simulink model "untitled4"  (R2025a)
settings: Solver=VariableStepAuto  StartTime=0.0  StopTime=10.0  RelTol=1e-3
libraries: fuzblock x1
settings Model: Creator=Win 11  LastModifiedBy=Win 11

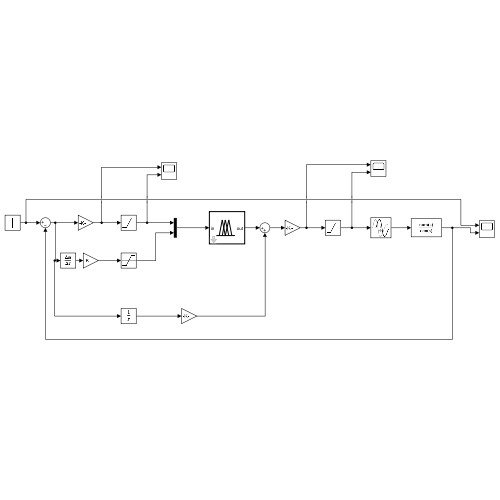
[thumbnail: Simulink's stored preview of the top-level diagram]
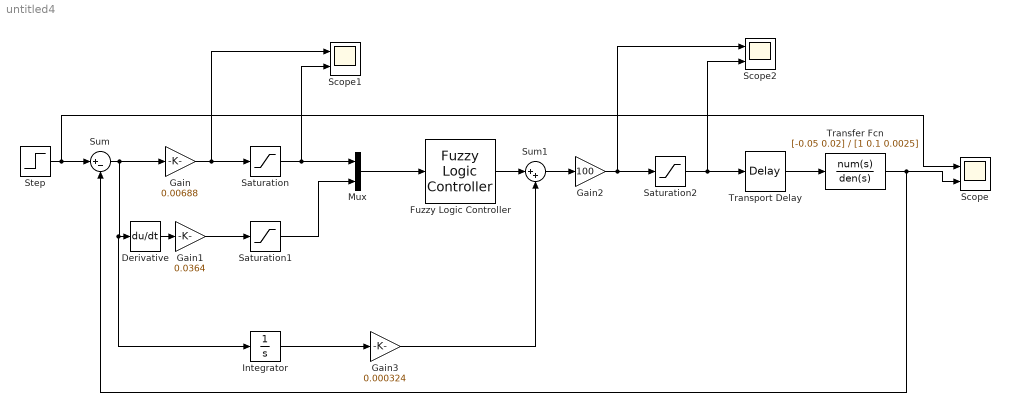
== system untitled4 ==
  Derivative : Derivative
  Fuzzy Logic Controller : fuzblock/Fuzzy Logic  Controller  FIS=fis  OutputSampleNumber=101  DataType=double  UseLookupTable=off  NumBreakpoints=10  FuzzifiedInputs=off  RuleFiringStrengths=off  RuleOutputs=off  AggregatedOutputs=off  SimulateUsing=Interpreted execution  OutOfRangeInputValueMessage=warning  NoRuleFiredMessage=warning  EmptyOutputFuzzySetMessage=warning
  Gain : Gain  Gain=0.00688
  Gain1 : Gain  Gain=0.0364
  Gain2 : Gain  Gain=100
  Gain3 : Gain  Gain=0.000324
  Integrator : Integrator
  Mux : Mux  Inputs=2
  Saturation : Saturate  UpperLimit=4  LowerLimit=-4
  Saturation1 : Saturate  UpperLimit=4  LowerLimit=-4
  Saturation2 : Saturate  UpperLimit=+2.2  LowerLimit=-2.2
  Scope : Scope  NumInputPorts=2
      settings: ActiveDisplayYMinimum=-0.140071912811771  ActiveDisplayYMaximum=1.1266746569790858
  Scope1 : Scope  NumInputPorts=2
      settings: ActiveDisplayYMinimum=-0.00087152164001610922  ActiveDisplayYMaximum=0.0078436947601449852
  Scope2 : Scope  NumInputPorts=2
      settings: ActiveDisplayYMinimum=-13.773649999999998  ActiveDisplayYMaximum=123.96285000000002  DataLoggingVariableName=ScopeData2
  Step : Step  SampleTime=0
  Sum : Sum  Inputs=|+-
  Sum1 : Sum  Inputs=|++
  Transfer Fcn : TransferFcn  Numerator=[-0.05 0.02]  Denominator=[1 0.1 0.0025]
  Transport Delay : TransportDelay  DelayTime=2
  wires:
  Step/1 -> Scope/1, Sum/1
  Gain/1 -> Scope1/1, Saturation/1
  Saturation/1 -> Scope1/2, Mux/1
  Saturation1/1 -> Mux/2
  Mux/1 -> Fuzzy Logic Controller/1
  Fuzzy Logic Controller/1 -> Sum1/1
  Sum1/1 -> Gain2/1
  Gain2/1 -> Scope2/1, Saturation2/1
  Saturation2/1 -> Scope2/2, Transport Delay/1
  Transport Delay/1 -> Transfer Fcn/1
  Transfer Fcn/1 -> Sum/2, Scope/2
  Integrator/1 -> Gain3/1
  Gain3/1 -> Sum1/2
  Gain1/1 -> Saturation1/1
  Derivative/1 -> Gain1/1
  Sum/1 -> Gain/1, Integrator/1, Derivative/1
